simulink model "sim_3_twolink_task_control"  (R2021a)
settings: Solver=VariableStepAuto  StartTime=0.0  StopTime=10.0  RelTol=1e-3
values from neighbouring files (symbols this model uses):
  b1 = 0.01    [sim_params.m]    (also in sim_params_force.m)
  b2 = 0.01    [sim_params.m]    (also in sim_params_force.m)
  D = [zeros(n); eye(n)]    [control_comparison_script.m]    (also in gen_twolink_ss.m = reshape([0.0,0.0,0.0,0.0,0.0,0.0,0.0,0.0],[4,2]))
  g = 9.80665    [sim_params.m]    (also in sim_params_force.m)
  Klqr = lqr(A,B,Q,R)    [control_comparison_script.m]
  Kpp = place(A,B,p)    [control_comparison_script.m]
  L1x = 0.3    [sim_params.m]    (also in sim_params_force.m)
  L1y = 0.050    (= 0.05)    [sim_params.m]    (also in sim_params_force.m)
  L1z = 0.05    [sim_params.m]    (also in sim_params_force.m)
  L2x = 0.15    [sim_params.m]    (also in sim_params_force.m = 0.3)
  L2y = 0.05    [sim_params.m]    (also in sim_params_force.m)
  L2z = 0.05    [sim_params.m]    (also in sim_params_force.m)
  m1 = m1*1.25    [control_comparison_script.m]    (also in sim_params.m = 2.775; sim_params_force.m = 2.775)
  m2 = m2*1.25    [control_comparison_script.m]    (also in sim_params.m = 1.3875; sim_params_force.m = 2.775)
  max_joint_torque1 = 20    [sim_params.m]    (also in sim_params_force.m)
  max_joint_torque2 = 10    [sim_params.m]    (also in sim_params_force.m = 20)
  theta1_0 = 0    [sim_params.m]    (also in sim_params_force.m = 1.57079632679)
  theta1_dot_0 = 0    [sim_params.m]    (also in sim_params_force.m)
  theta2_0 = 0    [sim_params.m]    (also in sim_params_force.m = -1.57079632679)
  theta2_dot_0 = 0    [sim_params.m]    (also in sim_params_force.m)
undefined symbols (not defined in the file or in its folder): Kslide, lambda, Levenberg, Marquardt, phi, sigbuilder_block, X, Y, Z
libraries: sm_lib x11, nesl_utility x10, simulink x8, pid_lib x6, robotmaniplib x3, robotcorelib x1
(part 1 of 2)
settings Model: Creator=Petronas-Tareq  LastModifiedBy=Petronas-Tareq

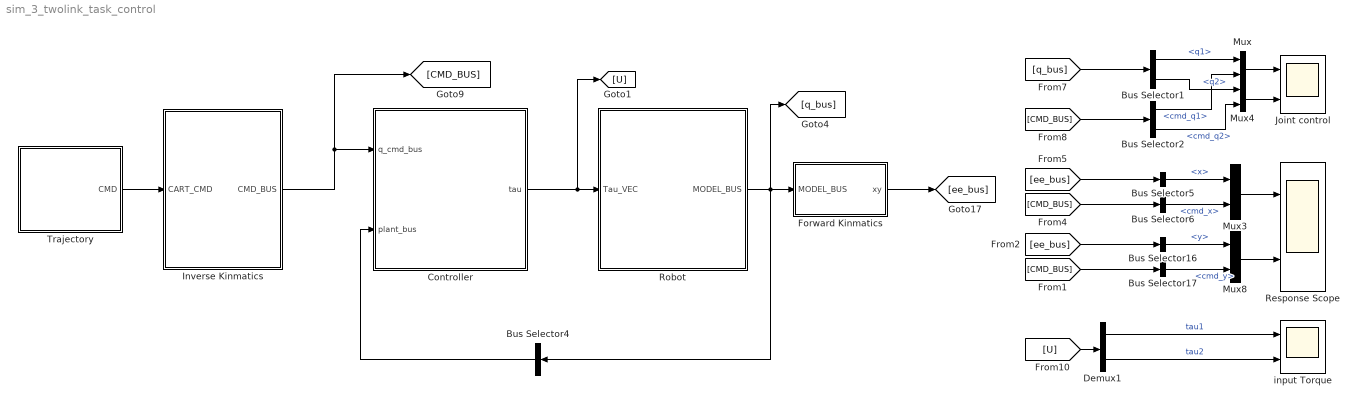
== system sim_3_twolink_task_control ==
  Bus Selector1 : BusSelector  OutputSignals=q1,q2
  Bus Selector16 : BusSelector  OutputSignals=y
  Bus Selector17 : BusSelector  OutputSignals=cmd_y
  Bus Selector2 : BusSelector  OutputSignals=cmd_q1,cmd_q2
  Bus Selector4 : BusSelector  OutputSignals=q1_dd,q2_dd,q1_d,q2_d,q1,q2  OutputAsBus=on
  Bus Selector5 : BusSelector  OutputSignals=x
  Bus Selector6 : BusSelector  OutputSignals=cmd_x
  Controller : Subsystem  Variant=on  VariantControlMode=label  LabelModeActiveChoice=PD_plus_gravity  PropagateVariantConditions=on
  Demux1 : Demux  Outputs=2
  Forward Kinmatics : Subsystem
  Inverse Kinmatics : Subsystem
  Joint control : Scope  NumInputPorts=2
  Mux{,3..4,8} (4 alike) : Mux  Inputs=2
  Response Scope : Scope  NumInputPorts=2
  Robot : Subsystem  Variant=on  VariantControlMode=label  LabelModeActiveChoice=Choice_1
  Trajectory : Subsystem  Variant=on  VariantControlMode=label  LabelModeActiveChoice=ramp
  input Torque : Scope  NumInputPorts=2
  wires:
  Trajectory/1(CMD) -> Inverse Kinmatics/1(CART_CMD)
  Robot/1(MODEL_BUS) -> Forward Kinmatics/1(MODEL_BUS), [q_bus], Bus Selector4/1
  Controller/1(tau) -> [U], Robot/1(Tau_VEC)
  Bus Selector4/1 -> Controller/2(plant_bus)
  Bus Selector2/1 -> Mux/2  "<cmd_q1>"
  Bus Selector1/2 -> Mux4/1  "<q2>"
  Mux4/1 -> Joint control/2
  [CMD_BUS] -> Bus Selector2/1
  Bus Selector1/1 -> Mux/1  "<q1>"
  Mux/1 -> Joint control/1
  Bus Selector2/2 -> Mux4/2  "<cmd_q2>"
  [q_bus] -> Bus Selector1/1
  Inverse Kinmatics/1(CMD_BUS) -> [CMD_BUS], Controller/1(q_cmd_bus)
  [ee_bus] -> Bus Selector5/1
  Bus Selector17/1 -> Mux8/2  "<cmd_y>"
  [U] -> Demux1/1
  [CMD_BUS] -> Bus Selector17/1
  Bus Selector16/1 -> Mux8/1  "<y>"
  Demux1/2 -> input Torque/2  "tau2"
  [ee_bus] -> Bus Selector16/1
  Demux1/1 -> input Torque/1  "tau1"
  Mux8/1 -> Response Scope/2
  Bus Selector6/1 -> Mux3/2  "<cmd_x>"
  [CMD_BUS] -> Bus Selector6/1
  Bus Selector5/1 -> Mux3/1  "<x>"
  Mux3/1 -> Response Scope/1
  Forward Kinmatics/1(xy) -> [ee_bus]

== system sim_3_twolink_task_control/Controller ==
  note: 1) Add Subsystem or Model blocks as valid variant choices.
      | 2) You cannot connect blocks at this level. At simulation, connectivity is automatically
      | determined, based on the active variant and port name matching.
  q_cmd_bus : Inport
  plant_bus : Inport  Port=2
  Incremental sliding mode Control : Subsystem  VariantControl=Sliding_mode_control
  "Inverse Dynamics control " : Subsystem  VariantControl=Inverse_dynamics_control
  LQR+D Control : Subsystem  VariantControl=LQR_D_control
  "PD-gravity Control " : Subsystem  VariantControl=PD_plus_gravity
  PID Control : Subsystem  VariantControl=PID_control
  Pole Placement+D Control : Subsystem  VariantControl=PolePlacement_D_control
  tau : Outport

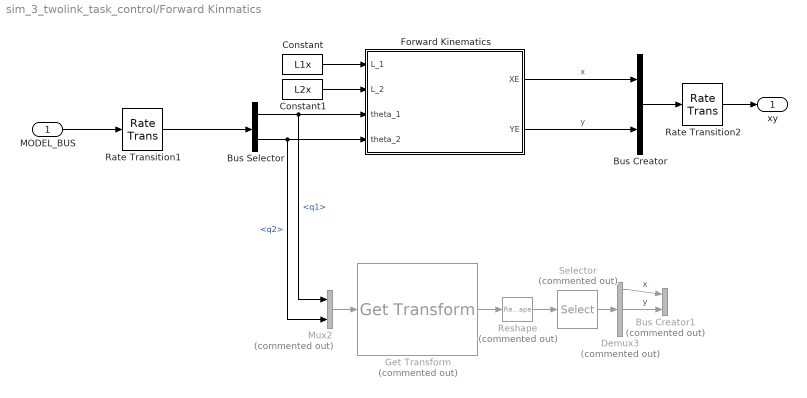
== system sim_3_twolink_task_control/Forward Kinmatics ==
  MODEL_BUS : Inport
  Bus Creator : BusCreator  Inputs=2
  Bus Creator1 : BusCreator  Commented=on  Inputs=2
  Bus Selector : BusSelector  OutputSignals=q1,q2
  Constant : Constant  Value=L1x
  Constant1 : Constant  Value=L2x
  Demux3 : Demux  Commented=on  Outputs=3
  Forward Kinematics : MATLAB Function  TreatAsAtomicUnit=on
  Get Transform : robotmaniplib/Get Transform  Commented=on  RigidBodyTree=RR_robot  SourceBody=end_effector  TargetBody=base  SimulateUsing=Interpreted execution
  Mux2 : Mux  Commented=on  Inputs=2
  Rate Transition1 : RateTransition  OutPortSampleTimeOpt=Inherit
  Rate Transition2 : RateTransition  OutPortSampleTimeOpt=Inherit
  Reshape : Reshape  Commented=on
  Selector : Selector  Commented=on  InputPortWidth=16  IndexOptions=Index vector (dialog)  Indices=[13:15]  OutputSizes=1
  xy : Outport
  wires:
  Forward Kinematics/2(YE) -> Bus Creator/2  "y"
  Forward Kinematics/1(XE) -> Bus Creator/1  "x"
  Bus Selector/1 -> Mux2/1, Forward Kinematics/3(theta_1)  "<q1>"
  MODEL_BUS/1 -> Rate Transition1/1
  Bus Selector/2 -> Mux2/2, Forward Kinematics/4(theta_2)  "<q2>"
  Constant/1 -> Forward Kinematics/1(L_1)
  Constant1/1 -> Forward Kinematics/2(L_2)
  Bus Creator/1 -> Rate Transition2/1
  Mux2/1 -> Get Transform/1
  Get Transform/1 -> Reshape/1
  Reshape/1 -> Selector/1
  Selector/1 -> Demux3/1
  Demux3/1 -> Bus Creator1/1  "x"
  Demux3/2 -> Bus Creator1/2  "y"
  Rate Transition2/1 -> xy/1
  Rate Transition1/1 -> Bus Selector/1

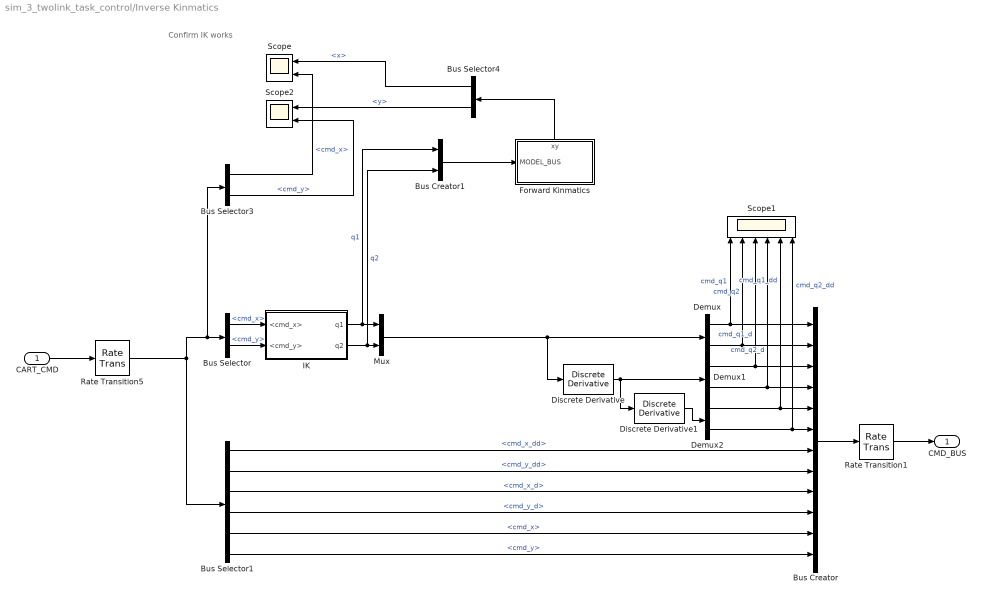
== system sim_3_twolink_task_control/Inverse Kinmatics ==
  note: Confirm IK works
  CART_CMD : Inport
  Bus Creator : BusCreator  Inputs=12
  Bus Creator1 : BusCreator  Inputs=2
  Bus Selector : BusSelector  OutputSignals=cmd_x,cmd_y
  Bus Selector1 : BusSelector  OutputSignals=cmd_x_dd,cmd_y_dd,cmd_x_d,cmd_y_d,cmd_x,cmd_y
  Bus Selector3 : BusSelector  OutputSignals=cmd_x,cmd_y
  Bus Selector4 : BusSelector  OutputSignals=x,y
  Demux : Demux  Outputs=2
  Demux1 : Demux  Outputs=2
  Demux2 : Demux  Outputs=2
  Discrete Derivative : simulink/Discrete/Discrete Derivative  gainval=1.0  ICPrevScaledInput=0.0  OutMin=[]  OutMax=[]  OutDataType=fixdt(1, 16)  OutScaling=2^-10  DoSatur=off
  Discrete Derivative1 : simulink/Discrete/Discrete Derivative  gainval=1.0  ICPrevScaledInput=0.0  OutMin=[]  OutMax=[]  OutDataType=fixdt(1, 16)  OutScaling=2^-10  DoSatur=off
  Forward Kinmatics : Subsystem
      settings: PortSchema="{\"entries\":[{\"content\":{\"sides\":[{\"content\":{\"connectorIds\":[\"In1\"]},\"type\":\"ConnectorPlacement.EquallySpacedRectSide\",\"uuid\":\"2c0f0405-b445-4922-82b0-9ed34ea6e343\"},{\"content\":{\"connectorIds\":[],\"side\":\"RIGHT\"},\"type\":\"ConnectorPlacement.EquallySpacedRectSide\",\"uuid\":\"91fea7c3-4850-470e-b524-5886f9b138cb\"},{\"content\":{\"connectorIds\":[\"Out1\"],\"side\":\"TOP\"},\"type\":\"ConnectorPlacement.EquallySpacedRectSide\",\"uuid\":\"51029b8b-093e-4a55-82a5-f93421c28d2e\"}]},\"type\":\"ConnectorPlacement.EquallySpacedConnector\",\"uuid\":\"843aee16-b8cd-4273-ac03-a5f22ed539be\"}],\"packageUris\":[\"http://schema.mathworks.com/mf0/Connector/R2020b\"],\"version\":\"1.0\"}"
  IK : Subsystem
  Mux : Mux  Inputs=2
  Rate Transition1 : RateTransition  OutPortSampleTimeOpt=Inherit
  Rate Transition5 : RateTransition  OutPortSampleTimeOpt=Inherit
  Scope : Scope  NumInputPorts=2
  Scope1 : Scope  NumInputPorts=6
  Scope2 : Scope  NumInputPorts=2
  CMD_BUS : Outport
  wires:
  Rate Transition5/1 -> Bus Selector3/1, Bus Selector/1, Bus Selector1/1
  Bus Creator/1 -> Rate Transition1/1
  Bus Selector1/1 -> Bus Creator/7  "<cmd_x_dd>"
  Bus Selector1/2 -> Bus Creator/8  "<cmd_y_dd>"
  Bus Selector1/3 -> Bus Creator/9  "<cmd_x_d>"
  Bus Selector1/4 -> Bus Creator/10  "<cmd_y_d>"
  Bus Selector1/5 -> Bus Creator/11  "<cmd_x>"
  Bus Selector1/6 -> Bus Creator/12  "<cmd_y>"
  Demux1/1 -> Scope1/3, Bus Creator/3  "cmd_q1_d"
  Demux2/2 -> Scope1/6, Bus Creator/6  "cmd_q2_dd"
  Demux1/2 -> Scope1/4, Bus Creator/4  "cmd_q2_d"
  Demux/1 -> Scope1/1, Bus Creator/1  "cmd_q1"
  Demux/2 -> Scope1/2, Bus Creator/2  "cmd_q2"
  Bus Selector/1 -> IK/1(<cmd_x>)  "<cmd_x>"
  Bus Selector/2 -> IK/2(<cmd_y>)  "<cmd_y>"
  IK/1(q1) -> Bus Creator1/1, Mux/1  "q1"
  IK/2(q2) -> Bus Creator1/2, Mux/2  "q2"
  Mux/1 -> Demux/1, Discrete Derivative/1
  Discrete Derivative/1 -> Demux1/1, Discrete Derivative1/1
  Demux2/1 -> Scope1/5, Bus Creator/5  "cmd_q1_dd"
  Discrete Derivative1/1 -> Demux2/1
  CART_CMD/1 -> Rate Transition5/1
  Rate Transition1/1 -> CMD_BUS/1
  Bus Creator1/1 -> Forward Kinmatics/1(MODEL_BUS)
  Forward Kinmatics/1(xy) -> Bus Selector4/1
  Bus Selector3/1 -> Scope/2  "<cmd_x>"
  Bus Selector4/1 -> Scope/1  "<x>"
  Bus Selector4/2 -> Scope2/1  "<y>"
  Bus Selector3/2 -> Scope2/2  "<cmd_y>"

== system sim_3_twolink_task_control/Robot ==
  note: 1) Add Subsystem or Model blocks as valid variant choices.
      | 2) You cannot connect blocks at this level. At simulation, connectivity is automatically
      | determined, based on the active variant and port name matching.
  Tau_VEC : Inport
  SIMSCAPE_MODEL : Subsystem  VariantControl=Choice_1
  SIMULINK_MODEL : Subsystem  VariantControl=Choice
  MODEL_BUS : Outport

== system sim_3_twolink_task_control/Trajectory ==
  note: 1) Add Subsystem or Model blocks as valid variant choices.
      | 2) You cannot connect blocks at this level. At simulation, connectivity is automatically
      | determined, based on the active variant and port name matching.
  Sinewave command : Subsystem  VariantControl=sinwave
  Step command : Subsystem  VariantControl=step
  ramp command : Subsystem  VariantControl=ramp
  CMD : Outport

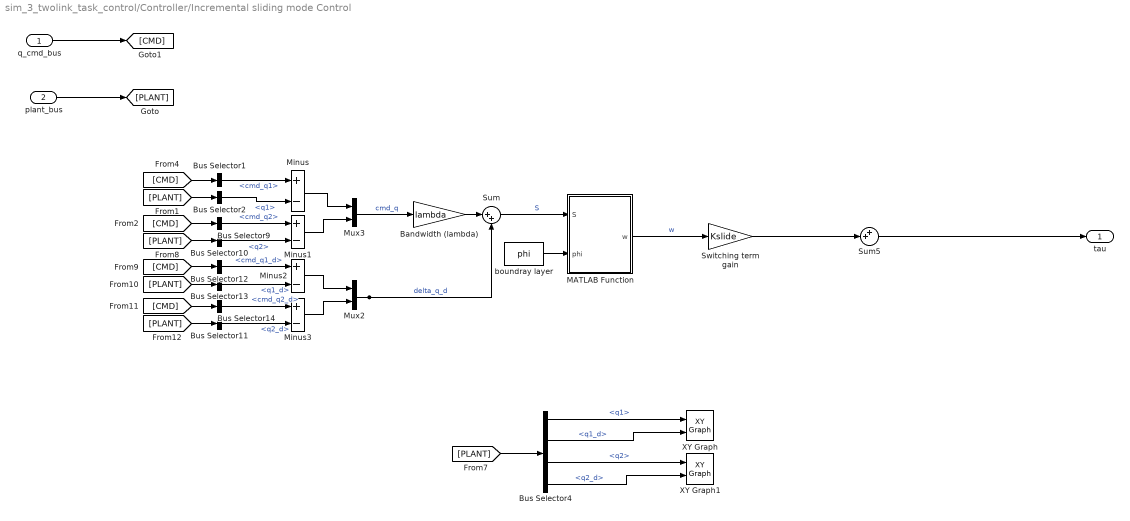
== system sim_3_twolink_task_control/Controller/Incremental sliding mode Control ==
  q_cmd_bus : Inport
  plant_bus : Inport  Port=2
  Bandwidth (lambda) : Gain  Gain=lambda
  Bus Selector1 : BusSelector  OutputSignals=cmd_q1
  Bus Selector10 : BusSelector  OutputSignals=q2
  Bus Selector11 : BusSelector  OutputSignals=q2_d
  Bus Selector12 : BusSelector  OutputSignals=cmd_q1_d
  Bus Selector13 : BusSelector  OutputSignals=q1_d
  Bus Selector14 : BusSelector  OutputSignals=cmd_q2_d
  Bus Selector2 : BusSelector  OutputSignals=q1
  Bus Selector4 : BusSelector  OutputSignals=q1,q1_d,q2,q2_d
  Bus Selector9 : BusSelector  OutputSignals=cmd_q2
  MATLAB Function : MATLAB Function  TreatAsAtomicUnit=on
  Minus{,1..3} (4 alike) : Sum  Inputs=+-
  Mux2 : Mux  Inputs=2
  Mux3 : Mux  Inputs=2
  Sum : Sum  Inputs=|++
  Sum5 : Sum  Inputs=++|
  Switching term gain : Gain  Gain=Kslide
  XY Graph : simulink/Sinks/XY Graph  xmin=-3  xmax=3  ymin=-3  ymax=3  st=-1
  XY Graph1 : simulink/Sinks/XY Graph  xmin=-3  xmax=3  ymin=-3  ymax=3  st=-1
  boundray layer : Constant  Value=phi
  tau : Outport
  wires:
  q_cmd_bus/1 -> [CMD]
  plant_bus/1 -> [PLANT]
  boundray layer/1 -> MATLAB Function/2(phi)
  [CMD] -> Bus Selector12/1
  Bus Selector1/1 -> Minus/1  "<cmd_q1>"
  [PLANT] -> Bus Selector13/1
  [PLANT] -> Bus Selector10/1
  [CMD] -> Bus Selector1/1
  Minus/1 -> Mux3/1
  [PLANT] -> Bus Selector11/1
  Minus3/1 -> Mux2/2
  [CMD] -> Bus Selector9/1
  Bus Selector12/1 -> Minus2/1  "<cmd_q1_d>"
  Bus Selector10/1 -> Minus1/2  "<q2>"
  Bus Selector2/1 -> Minus/2  "<q1>"
  Bus Selector9/1 -> Minus1/1  "<cmd_q2>"
  [PLANT] -> Bus Selector2/1
  Bus Selector11/1 -> Minus3/2  "<q2_d>"
  Bus Selector13/1 -> Minus2/2  "<q1_d>"
  Bus Selector14/1 -> Minus3/1  "<cmd_q2_d>"
  Minus2/1 -> Mux2/1
  [CMD] -> Bus Selector14/1
  Minus1/1 -> Mux3/2
  Sum/1 -> MATLAB Function/1(S)  "S"
  MATLAB Function/1(w) -> Switching term gain/1  "w"
  Switching term gain/1 -> Sum5/2
  Mux3/1 -> Bandwidth (lambda)/1  "cmd_q"
  Mux2/1 -> Sum/2  "delta_q_d"
  Bandwidth (lambda)/1 -> Sum/1
  Sum5/1 -> tau/1
  Bus Selector4/1 -> XY Graph/1  "<q1>"
  [PLANT] -> Bus Selector4/1
  Bus Selector4/2 -> XY Graph/2  "<q1_d>"
  Bus Selector4/3 -> XY Graph1/1  "<q2>"
  Bus Selector4/4 -> XY Graph1/2  "<q2_d>"

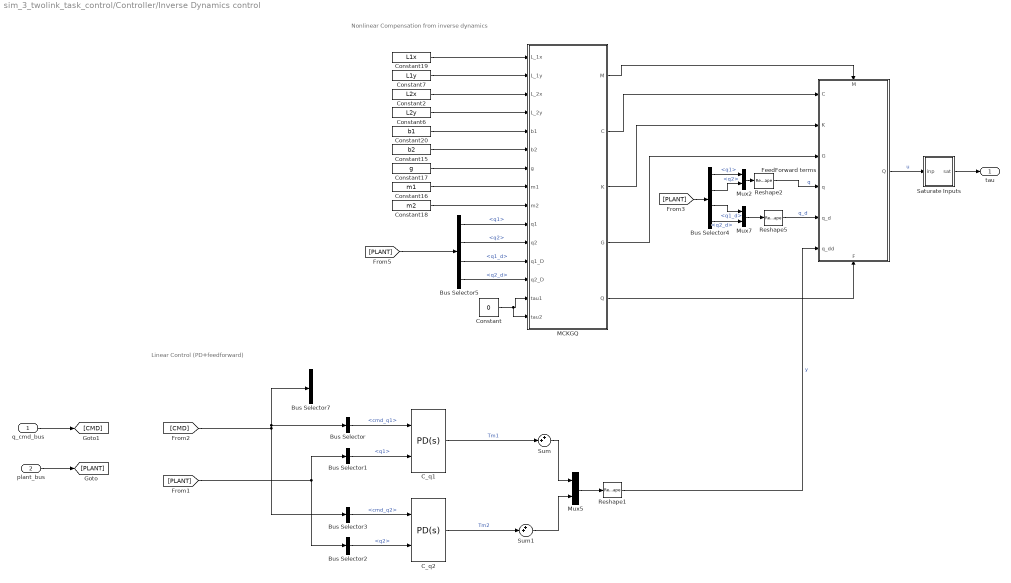
== system sim_3_twolink_task_control/Controller/Inverse Dynamics control  ==
  note: Nonlinear Compensation from inverse dynamics
  note: Linear Control (PD+feedforward)
  q_cmd_bus : Inport
  plant_bus : Inport  Port=2
  Bus Selector : BusSelector  OutputSignals=cmd_q1
  Bus Selector1 : BusSelector  OutputSignals=q1
  Bus Selector2 : BusSelector  OutputSignals=q2
  Bus Selector3 : BusSelector  OutputSignals=cmd_q2
  Bus Selector4 : BusSelector  OutputSignals=q1,q2,q1_d,q2_d
  Bus Selector5 : BusSelector  OutputSignals=q1,q2,q1_d,q2_d
  Bus Selector7 : BusSelector  OutputSignals=cmd_q1_dd,cmd_q2_dd
  C_q1 : pid_lib/PID Controller (2DOF)  Controller=PD  Form=Parallel  TimeDomain=Continuous-time  UseExternalTs=off  SampleTime=-1  IntegratorMethod=Forward Euler  FilterMethod=Forward Euler  ControllerParametersSource=internal  P=400  I=20  D=40  UseFilter=on  N=100  b=1  c=1  TunerSelectOption=Transfer Function Based (PID Tuner App)  InitialConditionSource=internal  InitialConditionForIntegrator=0  InitialConditionForFilter=0  DifferentiatorICPrevScaledInput=0  ExternalReset=none  TrackingMode=off  Kt=1  LimitOutput=on  SatLimitsSource=internal  UpperSaturationLimit=max_joint_torque1  LowerSaturationLimit=-max_joint_torque1  LinearizeAsGain=on  AntiWindupMode=none  Kb=1  POutMin=[]  POutMax=[]  IOutMin=[]  IOutMax=[]  DOutMin=[]  DOutMax=[]  NOutMin=[]  NOutMax=[]  bOutMin=[]  bOutMax=[]  cOutMin=[]  cOutMax=[]  SumOutMin=[]  SumOutMax=[]  SaturationOutMin=[]  SaturationOutMax=[]  PParamMin=[]  PParamMax=[]  IParamMin=[]  IParamMax=[]  DParamMin=[]  DParamMax=[]  NParamMin=[]  NParamMax=[]  bParamMin=[]  bParamMax=[]  cParamMin=[]  cParamMax=[]  KbParamMin=[]  KbParamMax=[]  KtParamMin=[]  KtParamMax=[]  KbOutMin=[]  KbOutMax=[]  KtOutMin=[]  KtOutMax=[]  IntegratorOutMin=[]  IntegratorOutMax=[]  FilterOutMin=[]  FilterOutMax=[]  SumI1OutMin=[]  SumI1OutMax=[]  SumI2OutMin=[]  SumI2OutMax=[]  SumI3OutMin=[]  SumI3OutMax=[]  SumI4OutMin=[]  SumI4OutMax=[]  SumDOutMin=[]  SumDOutMax=[]  Sum1OutMin=[]  Sum1OutMax=[]  Sum2OutMin=[]  Sum2OutMax=[]  Sum3OutMin=[]  Sum3OutMax=[]  DifferentiatorOutMin=[]  DifferentiatorOutMax=[]  FilterDiffOutCoefMin=[]  FilterDiffOutCoefMax=[]  ReciprocalOutMin=[]  ReciprocalOutMax=[]  SumDenOutMin=[]  SumDenOutMax=[]  SumNumOutMin=[]  SumNumOutMax=[]  DivideOutMin=[]  DivideOutMax=[]  UdiffTsProdOutMin=[]  UdiffTsProdOutMax=[]  NTsProdOutMin=[]  NTsProdOutMax=[]  UintegralTsProdOutMin=[]  UintegralTsProdOutMax=[]  UngainTsProdOutMin=[]  UngainTsProdOutMax=[]  IntegratorContinuousStateAttributes=''  IntegratorStateMustResolveToSignalObject=off  IntegratorRTWStateStorageClass=Auto  FilterContinuousStateAttributes=''  FilterStateMustResolveToSignalObject=off  FilterRTWStateStorageClass=Auto  ParallelPVariant=InternalParameters  IdealPVariant=Disabled  IVariant=Disabled  DVariant=InternalParameters  bVariant=InternalParameters  cVariant=InternalParameters  IntegratorVariant=Disabled  SatVariant=Enabled  AWVariant=Disabled  PCopyVariant=Disabled  TRVariant=Disabled  FdbkBlocksVariant=Forward  IdealPFdbkVariant=Disabled  SatFdbkVariant=Disabled  DerivativeFilterVariant=ContFilter  NVariant=InternalParameters  NCopyVariant=Disabled  FilterICVariant=InternalICsFilter  IntegratorICVariant=Disabled  ExternalResetVariant=Disabled  TRSumVariant=Passthrough  SumFdbkVariant=Disabled  SumVariant=Sum_PD  TsampFilterVariant=InternalTs  TsampNgainVariant=Passthrough  TsampIntegralVariant=Disabled_SignalSpec  ExternalSaturationOutDataTypeStr=Inherit: Same as second input
      settings: SourceProductBaseCode=SL
  C_q2 : pid_lib/PID Controller (2DOF)  Controller=PD  Form=Parallel  TimeDomain=Continuous-time  UseExternalTs=off  SampleTime=-1  IntegratorMethod=Forward Euler  FilterMethod=Forward Euler  ControllerParametersSource=internal  P=200  I=20  D=35  UseFilter=on  N=100  b=1  c=1  TunerSelectOption=Transfer Function Based (PID Tuner App)  InitialConditionSource=internal  InitialConditionForIntegrator=0  InitialConditionForFilter=0  DifferentiatorICPrevScaledInput=0  ExternalReset=none  TrackingMode=off  Kt=1  LimitOutput=on  SatLimitsSource=internal  UpperSaturationLimit=max_joint_torque2  LowerSaturationLimit=-max_joint_torque2  LinearizeAsGain=on  AntiWindupMode=none  Kb=1  POutMin=[]  POutMax=[]  IOutMin=[]  IOutMax=[]  DOutMin=[]  DOutMax=[]  NOutMin=[]  NOutMax=[]  bOutMin=[]  bOutMax=[]  cOutMin=[]  cOutMax=[]  SumOutMin=[]  SumOutMax=[]  SaturationOutMin=[]  SaturationOutMax=[]  PParamMin=[]  PParamMax=[]  IParamMin=[]  IParamMax=[]  DParamMin=[]  DParamMax=[]  NParamMin=[]  NParamMax=[]  bParamMin=[]  bParamMax=[]  cParamMin=[]  cParamMax=[]  KbParamMin=[]  KbParamMax=[]  KtParamMin=[]  KtParamMax=[]  KbOutMin=[]  KbOutMax=[]  KtOutMin=[]  KtOutMax=[]  IntegratorOutMin=[]  IntegratorOutMax=[]  FilterOutMin=[]  FilterOutMax=[]  SumI1OutMin=[]  SumI1OutMax=[]  SumI2OutMin=[]  SumI2OutMax=[]  SumI3OutMin=[]  SumI3OutMax=[]  SumI4OutMin=[]  SumI4OutMax=[]  SumDOutMin=[]  SumDOutMax=[]  Sum1OutMin=[]  Sum1OutMax=[]  Sum2OutMin=[]  Sum2OutMax=[]  Sum3OutMin=[]  Sum3OutMax=[]  DifferentiatorOutMin=[]  DifferentiatorOutMax=[]  FilterDiffOutCoefMin=[]  FilterDiffOutCoefMax=[]  ReciprocalOutMin=[]  ReciprocalOutMax=[]  SumDenOutMin=[]  SumDenOutMax=[]  SumNumOutMin=[]  SumNumOutMax=[]  DivideOutMin=[]  DivideOutMax=[]  UdiffTsProdOutMin=[]  UdiffTsProdOutMax=[]  NTsProdOutMin=[]  NTsProdOutMax=[]  UintegralTsProdOutMin=[]  UintegralTsProdOutMax=[]  UngainTsProdOutMin=[]  UngainTsProdOutMax=[]  IntegratorContinuousStateAttributes=''  IntegratorStateMustResolveToSignalObject=off  IntegratorRTWStateStorageClass=Auto  FilterContinuousStateAttributes=''  FilterStateMustResolveToSignalObject=off  FilterRTWStateStorageClass=Auto  ParallelPVariant=InternalParameters  IdealPVariant=Disabled  IVariant=Disabled  DVariant=InternalParameters  bVariant=InternalParameters  cVariant=InternalParameters  IntegratorVariant=Disabled  SatVariant=Enabled  AWVariant=Disabled  PCopyVariant=Disabled  TRVariant=Disabled  FdbkBlocksVariant=Forward  IdealPFdbkVariant=Disabled  SatFdbkVariant=Disabled  DerivativeFilterVariant=ContFilter  NVariant=InternalParameters  NCopyVariant=Disabled  FilterICVariant=InternalICsFilter  IntegratorICVariant=Disabled  ExternalResetVariant=Disabled  TRSumVariant=Passthrough  SumFdbkVariant=Disabled  SumVariant=Sum_PD  TsampFilterVariant=InternalTs  TsampNgainVariant=Passthrough  TsampIntegralVariant=Disabled_SignalSpec  ExternalSaturationOutDataTypeStr=Inherit: Same as second input
      settings: SourceProductBaseCode=SL
  Constant : Constant  Value=0
  Constant15 : Constant  Value=b2
  Constant16 : Constant  Value=m1
  Constant17 : Constant  Value=g
  Constant18 : Constant  Value=m2
  Constant19 : Constant  Value=L1x
  Constant2 : Constant  Value=L2x
  Constant20 : Constant  Value=b1
  Constant6 : Constant  Value=L2y
  Constant7 : Constant  Value=L1y
  FeedForward terms : Subsystem
      settings: PortSchema="{\"entries\":[{\"content\":{\"sides\":[{\"content\":{\"connectorIds\":[\"In1\",\"In2\",\"In3\",\"In4\",\"In5\",\"In6\"]},\"type\":\"ConnectorPlacement.EquallySpacedRectSide\",\"uuid\":\"236e7a2f-027c-4887-b3e9-bc0e11a59ec6\"},{\"content\":{\"connectorIds\":[\"Out1\"],\"side\":\"RIGHT\"},\"type\":\"ConnectorPlacement.EquallySpacedRectSide\",\"uuid\":\"0b727d96-7650-4ea0-95ac-5fb1bad7af10\"},{\"content\":{\"connectorIds\":[\"In7\"],\"side\":\"TOP\"},\"type\":\"ConnectorPlacement.EquallySpacedRectSide\",\"uuid\":\"19d9c8c6-ae7e-49b4-b718-472bd3040569\"},{\"content\":{\"connectorIds\":[\"In8\"],\"side\":\"BOTTOM\"},\"type\":\"ConnectorPlacement.EquallySpacedRectSide\",\"uuid\":\"734f5953-872d-4718-8798-69ea98da43e1\"}]},\"type\":\"ConnectorPlacement.EquallySpacedConnector\",\"uuid\":\"f4b93fea-e2dd-47f1-bf2a-cf2dec03adb9\"}],\"packageUris\":[\"http://schema.mathworks.com/mf0/Connector/R2020b\"],\"version\":\"1.0\"}"
  MCKGQ : MATLAB Function  TreatAsAtomicUnit=on
  Mux2 : Mux  Inputs=2
  Mux5 : Mux  Inputs=2
  Mux7 : Mux  Inputs=2
  Reshape1 : Reshape  OutputDimensionality=Column vector (2-D)
  Reshape2 : Reshape  OutputDimensionality=Column vector (2-D)
  Reshape5 : Reshape  OutputDimensionality=Column vector (2-D)
  Saturate Inputs : Subsystem
  Sum : Sum  Inputs=++|
  Sum1 : Sum  Inputs=++|
  tau : Outport
  wires:
  C_q1/1 -> Sum/2  "Tm1"
  q_cmd_bus/1 -> [CMD]
  plant_bus/1 -> [PLANT]
  Bus Selector2/1 -> C_q2/2  "<q2>"
  Bus Selector3/1 -> C_q2/1  "<cmd_q2>"
  Bus Selector1/1 -> C_q1/2  "<q1>"
  Bus Selector/1 -> C_q1/1  "<cmd_q1>"
  [PLANT] -> Bus Selector1/1, Bus Selector2/1
  Bus Selector5/4 -> MCKGQ/13(q2_D)  "<q2_d>"
  Bus Selector5/3 -> MCKGQ/12(q1_D)  "<q1_d>"
  Bus Selector5/1 -> MCKGQ/10(q1)  "<q1>"
  [PLANT] -> Bus Selector5/1
  Bus Selector5/2 -> MCKGQ/11(q2)  "<q2>"
  Mux5/1 -> Reshape1/1
  FeedForward terms/1(Q) -> Saturate Inputs/1(inp)  "u"
  [CMD] -> Bus Selector7/1, Bus Selector/1, Bus Selector3/1
  Sum/1 -> Mux5/1
  C_q2/1 -> Sum1/2  "Tm2"
  Sum1/1 -> Mux5/2
  [PLANT] -> Bus Selector4/1
  Bus Selector4/3 -> Mux7/1  "<q1_d>"
  Bus Selector4/4 -> Mux7/2  "<q2_d>"
  Mux7/1 -> Reshape5/1
  Reshape5/1 -> FeedForward terms/5(q_d)  "q_d"
  Reshape1/1 -> FeedForward terms/6(q_dd)  "y"
  MCKGQ/2(C) -> FeedForward terms/1(C)
  MCKGQ/3(K) -> FeedForward terms/2(K)
  MCKGQ/4(G) -> FeedForward terms/3(G)
  Bus Selector4/1 -> Mux2/1  "<q1>"
  Bus Selector4/2 -> Mux2/2  "<q2>"
  Mux2/1 -> Reshape2/1
  Reshape2/1 -> FeedForward terms/4(q)  "q"
  MCKGQ/5(Q) -> FeedForward terms/8(F)
  Constant/1 -> MCKGQ/14(tau1), MCKGQ/15(tau2)
  MCKGQ/1(M) -> FeedForward terms/7(M)
  Constant7/1 -> MCKGQ/2(L_1y)
  Constant2/1 -> MCKGQ/3(L_2x)
  Constant6/1 -> MCKGQ/4(L_2y)
  Constant20/1 -> MCKGQ/5(b1)
  Constant15/1 -> MCKGQ/6(b2)
  Constant17/1 -> MCKGQ/7(g)
  Constant16/1 -> MCKGQ/8(m1)
  Constant18/1 -> MCKGQ/9(m2)
  Constant19/1 -> MCKGQ/1(L_1x)
  Saturate Inputs/1(sat) -> tau/1

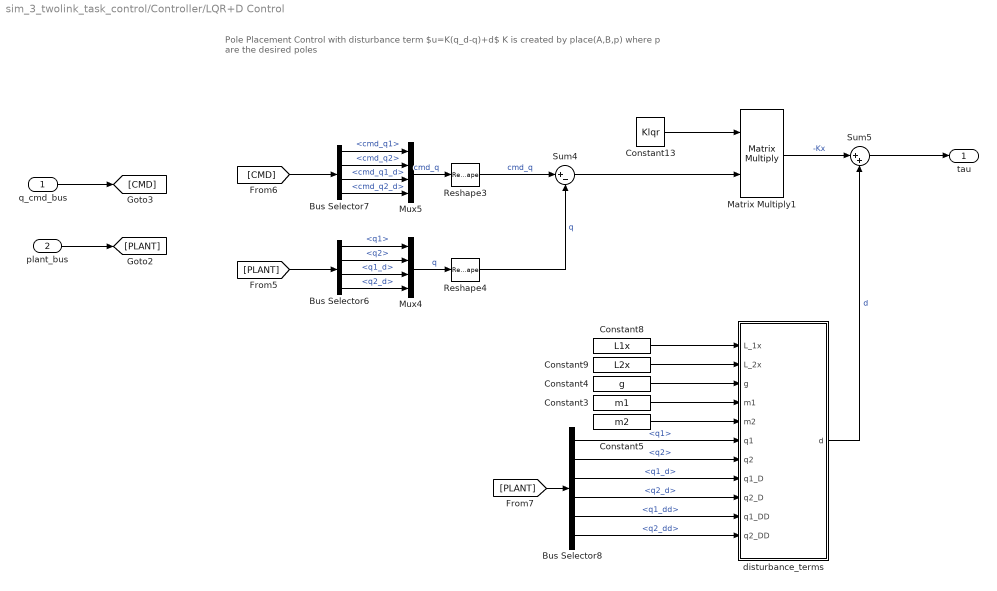
== system sim_3_twolink_task_control/Controller/LQR+D Control ==
  note: Pole Placement Control with disturbance term
      | $u=K(q_d-q)+d$
      | K is created by place(A,B,p) where p are the desired poles
  q_cmd_bus : Inport
  plant_bus : Inport  Port=2
  Bus Selector6 : BusSelector  OutputSignals=q1,q2,q1_d,q2_d
  Bus Selector7 : BusSelector  OutputSignals=cmd_q1,cmd_q2,cmd_q1_d,cmd_q2_d
  Bus Selector8 : BusSelector  OutputSignals=q1,q2,q1_d,q2_d,q1_dd,q2_dd
  Constant13 : Constant  Value=Klqr  VectorParams1D=off
  Constant3 : Constant  Value=m1
  Constant4 : Constant  Value=g
  Constant5 : Constant  Value=m2
  Constant8 : Constant  Value=L1x
  Constant9 : Constant  Value=L2x
  Matrix Multiply1 : Product  Multiplication=Matrix(*)
  Mux4 : Mux
  Mux5 : Mux
  Reshape3 : Reshape  OutputDimensionality=Column vector (2-D)
  Reshape4 : Reshape  OutputDimensionality=Column vector (2-D)
  Sum4 : Sum  Inputs=|+-
  Sum5 : Sum  Inputs=|++
  disturbance_terms : MATLAB Function  TreatAsAtomicUnit=on
  tau : Outport
  wires:
  Bus Selector6/2 -> Mux4/2  "<q2>"
  Bus Selector6/1 -> Mux4/1  "<q1>"
  Mux4/1 -> Reshape4/1  "q"
  q_cmd_bus/1 -> [CMD]
  plant_bus/1 -> [PLANT]
  Mux5/1 -> Reshape3/1  "cmd_q"
  Bus Selector6/3 -> Mux4/3  "<q1_d>"
  [PLANT] -> Bus Selector6/1
  Bus Selector6/4 -> Mux4/4  "<q2_d>"
  Reshape3/1 -> Sum4/1  "cmd_q"
  Reshape4/1 -> Sum4/2  "q"
  Matrix Multiply1/1 -> Sum5/1  "-Kx"
  Sum4/1 -> Matrix Multiply1/2
  Bus Selector7/1 -> Mux5/1  "<cmd_q1>"
  Bus Selector7/2 -> Mux5/2  "<cmd_q2>"
  Bus Selector7/3 -> Mux5/3  "<cmd_q1_d>"
  Constant13/1 -> Matrix Multiply1/1
  Bus Selector7/4 -> Mux5/4  "<cmd_q2_d>"
  [CMD] -> Bus Selector7/1
  Sum5/1 -> tau/1
  disturbance_terms/1(d) -> Sum5/2  "d"
  [PLANT] -> Bus Selector8/1
  Bus Selector8/1 -> disturbance_terms/6(q1)  "<q1>"
  Bus Selector8/2 -> disturbance_terms/7(q2)  "<q2>"
  Bus Selector8/3 -> disturbance_terms/8(q1_D)  "<q1_d>"
  Bus Selector8/4 -> disturbance_terms/9(q2_D)  "<q2_d>"
  Bus Selector8/5 -> disturbance_terms/10(q1_DD)  "<q1_dd>"
  Bus Selector8/6 -> disturbance_terms/11(q2_DD)  "<q2_dd>"
  Constant8/1 -> disturbance_terms/1(L_1x)
  Constant9/1 -> disturbance_terms/2(L_2x)
  Constant4/1 -> disturbance_terms/3(g)
  Constant3/1 -> disturbance_terms/4(m1)
  Constant5/1 -> disturbance_terms/5(m2)

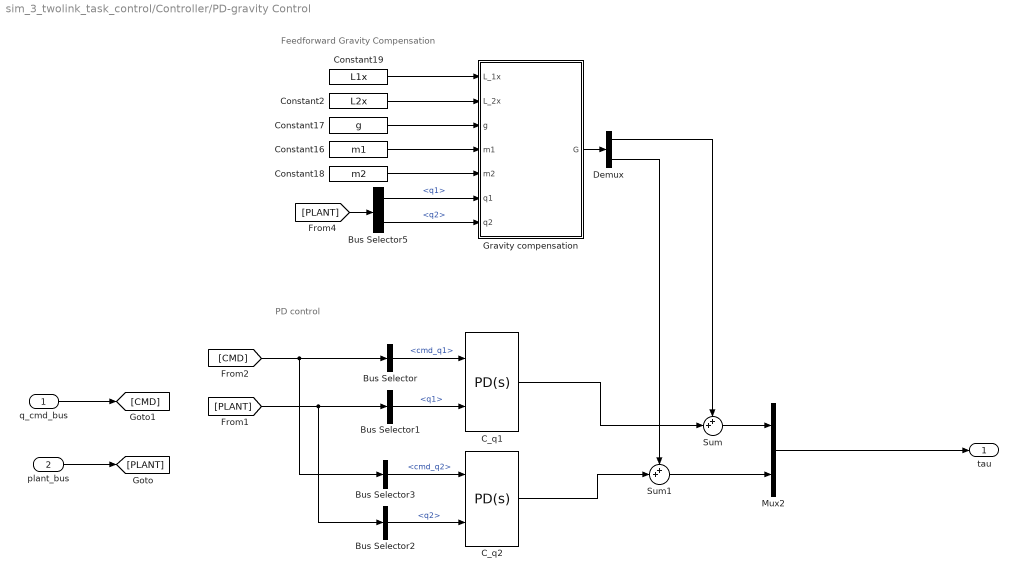
== system sim_3_twolink_task_control/Controller/PD-gravity Control  ==
  note: Feedforward Gravity Compensation
  note: PD control
  q_cmd_bus : Inport
  plant_bus : Inport  Port=2
  Bus Selector : BusSelector  OutputSignals=cmd_q1
  Bus Selector1 : BusSelector  OutputSignals=q1
  Bus Selector2 : BusSelector  OutputSignals=q2
  Bus Selector3 : BusSelector  OutputSignals=cmd_q2
  Bus Selector5 : BusSelector  OutputSignals=q1,q2
  C_q1 : pid_lib/PID Controller (2DOF)  Controller=PD  Form=Parallel  TimeDomain=Continuous-time  UseExternalTs=off  SampleTime=-1  IntegratorMethod=Forward Euler  FilterMethod=Forward Euler  ControllerParametersSource=internal  P=15  I=15  D=3  UseFilter=on  N=100  b=1  c=1  TunerSelectOption=Transfer Function Based (PID Tuner App)  InitialConditionSource=internal  InitialConditionForIntegrator=0  InitialConditionForFilter=0  DifferentiatorICPrevScaledInput=0  ExternalReset=none  TrackingMode=off  Kt=1  LimitOutput=off  SatLimitsSource=internal  UpperSaturationLimit=max_joint_torque1  LowerSaturationLimit=-max_joint_torque1  LinearizeAsGain=on  AntiWindupMode=none  Kb=1  POutMin=[]  POutMax=[]  IOutMin=[]  IOutMax=[]  DOutMin=[]  DOutMax=[]  NOutMin=[]  NOutMax=[]  bOutMin=[]  bOutMax=[]  cOutMin=[]  cOutMax=[]  SumOutMin=[]  SumOutMax=[]  SaturationOutMin=[]  SaturationOutMax=[]  PParamMin=[]  PParamMax=[]  IParamMin=[]  IParamMax=[]  DParamMin=[]  DParamMax=[]  NParamMin=[]  NParamMax=[]  bParamMin=[]  bParamMax=[]  cParamMin=[]  cParamMax=[]  KbParamMin=[]  KbParamMax=[]  KtParamMin=[]  KtParamMax=[]  KbOutMin=[]  KbOutMax=[]  KtOutMin=[]  KtOutMax=[]  IntegratorOutMin=[]  IntegratorOutMax=[]  FilterOutMin=[]  FilterOutMax=[]  SumI1OutMin=[]  SumI1OutMax=[]  SumI2OutMin=[]  SumI2OutMax=[]  SumI3OutMin=[]  SumI3OutMax=[]  SumI4OutMin=[]  SumI4OutMax=[]  SumDOutMin=[]  SumDOutMax=[]  Sum1OutMin=[]  Sum1OutMax=[]  Sum2OutMin=[]  Sum2OutMax=[]  Sum3OutMin=[]  Sum3OutMax=[]  DifferentiatorOutMin=[]  DifferentiatorOutMax=[]  FilterDiffOutCoefMin=[]  FilterDiffOutCoefMax=[]  ReciprocalOutMin=[]  ReciprocalOutMax=[]  SumDenOutMin=[]  SumDenOutMax=[]  SumNumOutMin=[]  SumNumOutMax=[]  DivideOutMin=[]  DivideOutMax=[]  UdiffTsProdOutMin=[]  UdiffTsProdOutMax=[]  NTsProdOutMin=[]  NTsProdOutMax=[]  UintegralTsProdOutMin=[]  UintegralTsProdOutMax=[]  UngainTsProdOutMin=[]  UngainTsProdOutMax=[]  IntegratorContinuousStateAttributes=''  IntegratorStateMustResolveToSignalObject=off  IntegratorRTWStateStorageClass=Auto  FilterContinuousStateAttributes=''  FilterStateMustResolveToSignalObject=off  FilterRTWStateStorageClass=Auto  ParallelPVariant=InternalParameters  IdealPVariant=Disabled  IVariant=Disabled  DVariant=InternalParameters  bVariant=InternalParameters  cVariant=InternalParameters  IntegratorVariant=Disabled  SatVariant=Disabled  AWVariant=Disabled  PCopyVariant=Disabled  TRVariant=Disabled  FdbkBlocksVariant=Forward  IdealPFdbkVariant=Disabled  SatFdbkVariant=Disabled  DerivativeFilterVariant=ContFilter  NVariant=InternalParameters  NCopyVariant=Disabled  FilterICVariant=InternalICsFilter  IntegratorICVariant=Disabled  ExternalResetVariant=Disabled  TRSumVariant=Passthrough  SumFdbkVariant=Disabled  SumVariant=Sum_PD  TsampFilterVariant=InternalTs  TsampNgainVariant=Passthrough  TsampIntegralVariant=Disabled_SignalSpec  ExternalSaturationOutDataTypeStr=Inherit: Same as second input
      settings: SourceProductBaseCode=SL
  C_q2 : pid_lib/PID Controller (2DOF)  Controller=PD  Form=Parallel  TimeDomain=Continuous-time  UseExternalTs=off  SampleTime=-1  IntegratorMethod=Forward Euler  FilterMethod=Forward Euler  ControllerParametersSource=internal  P=7  I=5  D=0.8  UseFilter=on  N=100  b=1  c=1  TunerSelectOption=Transfer Function Based (PID Tuner App)  InitialConditionSource=internal  InitialConditionForIntegrator=0  InitialConditionForFilter=0  DifferentiatorICPrevScaledInput=0  ExternalReset=none  TrackingMode=off  Kt=1  LimitOutput=off  SatLimitsSource=internal  UpperSaturationLimit=max_joint_torque2  LowerSaturationLimit=-max_joint_torque2  LinearizeAsGain=on  AntiWindupMode=none  Kb=1  POutMin=[]  POutMax=[]  IOutMin=[]  IOutMax=[]  DOutMin=[]  DOutMax=[]  NOutMin=[]  NOutMax=[]  bOutMin=[]  bOutMax=[]  cOutMin=[]  cOutMax=[]  SumOutMin=[]  SumOutMax=[]  SaturationOutMin=[]  SaturationOutMax=[]  PParamMin=[]  PParamMax=[]  IParamMin=[]  IParamMax=[]  DParamMin=[]  DParamMax=[]  NParamMin=[]  NParamMax=[]  bParamMin=[]  bParamMax=[]  cParamMin=[]  cParamMax=[]  KbParamMin=[]  KbParamMax=[]  KtParamMin=[]  KtParamMax=[]  KbOutMin=[]  KbOutMax=[]  KtOutMin=[]  KtOutMax=[]  IntegratorOutMin=[]  IntegratorOutMax=[]  FilterOutMin=[]  FilterOutMax=[]  SumI1OutMin=[]  SumI1OutMax=[]  SumI2OutMin=[]  SumI2OutMax=[]  SumI3OutMin=[]  SumI3OutMax=[]  SumI4OutMin=[]  SumI4OutMax=[]  SumDOutMin=[]  SumDOutMax=[]  Sum1OutMin=[]  Sum1OutMax=[]  Sum2OutMin=[]  Sum2OutMax=[]  Sum3OutMin=[]  Sum3OutMax=[]  DifferentiatorOutMin=[]  DifferentiatorOutMax=[]  FilterDiffOutCoefMin=[]  FilterDiffOutCoefMax=[]  ReciprocalOutMin=[]  ReciprocalOutMax=[]  SumDenOutMin=[]  SumDenOutMax=[]  SumNumOutMin=[]  SumNumOutMax=[]  DivideOutMin=[]  DivideOutMax=[]  UdiffTsProdOutMin=[]  UdiffTsProdOutMax=[]  NTsProdOutMin=[]  NTsProdOutMax=[]  UintegralTsProdOutMin=[]  UintegralTsProdOutMax=[]  UngainTsProdOutMin=[]  UngainTsProdOutMax=[]  IntegratorContinuousStateAttributes=''  IntegratorStateMustResolveToSignalObject=off  IntegratorRTWStateStorageClass=Auto  FilterContinuousStateAttributes=''  FilterStateMustResolveToSignalObject=off  FilterRTWStateStorageClass=Auto  ParallelPVariant=InternalParameters  IdealPVariant=Disabled  IVariant=Disabled  DVariant=InternalParameters  bVariant=InternalParameters  cVariant=InternalParameters  IntegratorVariant=Disabled  SatVariant=Disabled  AWVariant=Disabled  PCopyVariant=Disabled  TRVariant=Disabled  FdbkBlocksVariant=Forward  IdealPFdbkVariant=Disabled  SatFdbkVariant=Disabled  DerivativeFilterVariant=ContFilter  NVariant=InternalParameters  NCopyVariant=Disabled  FilterICVariant=InternalICsFilter  IntegratorICVariant=Disabled  ExternalResetVariant=Disabled  TRSumVariant=Passthrough  SumFdbkVariant=Disabled  SumVariant=Sum_PD  TsampFilterVariant=InternalTs  TsampNgainVariant=Passthrough  TsampIntegralVariant=Disabled_SignalSpec  ExternalSaturationOutDataTypeStr=Inherit: Same as second input
      settings: SourceProductBaseCode=SL
  Constant16 : Constant  Value=m1
  Constant17 : Constant  Value=g
  Constant18 : Constant  Value=m2
  Constant19 : Constant  Value=L1x
  Constant2 : Constant  Value=L2x
  Demux : Demux  Outputs=2
  Gravity compensation : MATLAB Function  TreatAsAtomicUnit=on
  Mux2 : Mux  Inputs=2
  Sum : Sum  Inputs=++|
  Sum1 : Sum  Inputs=++|
  tau : Outport
  wires:
  Sum/1 -> Mux2/1
  Sum1/1 -> Mux2/2
  q_cmd_bus/1 -> [CMD]
  plant_bus/1 -> [PLANT]
  Bus Selector5/1 -> Gravity compensation/6(q1)  "<q1>"
  [PLANT] -> Bus Selector5/1
  Bus Selector5/2 -> Gravity compensation/7(q2)  "<q2>"
  Gravity compensation/1(G) -> Demux/1
  Demux/1 -> Sum/1
  Demux/2 -> Sum1/1
  C_q2/1 -> Sum1/2
  [CMD] -> Bus Selector3/1, Bus Selector/1
  [PLANT] -> Bus Selector2/1, Bus Selector1/1
  Bus Selector1/1 -> C_q1/2  "<q1>"
  Bus Selector2/1 -> C_q2/2  "<q2>"
  Bus Selector3/1 -> C_q2/1  "<cmd_q2>"
  Bus Selector/1 -> C_q1/1  "<cmd_q1>"
  C_q1/1 -> Sum/2
  Constant19/1 -> Gravity compensation/1(L_1x)
  Constant2/1 -> Gravity compensation/2(L_2x)
  Constant17/1 -> Gravity compensation/3(g)
  Constant16/1 -> Gravity compensation/4(m1)
  Constant18/1 -> Gravity compensation/5(m2)
  Mux2/1 -> tau/1

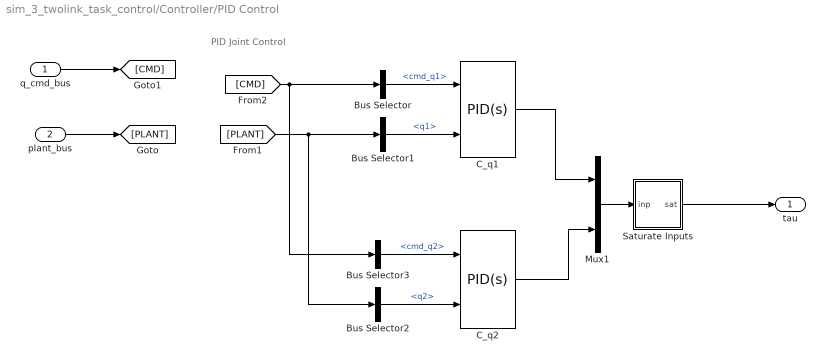
== system sim_3_twolink_task_control/Controller/PID Control ==
  note: PID Joint Control
  q_cmd_bus : Inport
  plant_bus : Inport  Port=2
  Bus Selector : BusSelector  OutputSignals=cmd_q1
  Bus Selector1 : BusSelector  OutputSignals=q1
  Bus Selector2 : BusSelector  OutputSignals=q2
  Bus Selector3 : BusSelector  OutputSignals=cmd_q2
  C_q1 : pid_lib/PID Controller (2DOF)  Controller=PID  Form=Parallel  TimeDomain=Continuous-time  UseExternalTs=off  SampleTime=-1  IntegratorMethod=Forward Euler  FilterMethod=Forward Euler  ControllerParametersSource=internal  P=30  I=20  D=2.5  UseFilter=on  N=100  b=1  c=1  TunerSelectOption=Transfer Function Based (PID Tuner App)  InitialConditionSource=internal  InitialConditionForIntegrator=0  InitialConditionForFilter=0  DifferentiatorICPrevScaledInput=0  ExternalReset=none  TrackingMode=off  Kt=1  LimitOutput=off  SatLimitsSource=internal  UpperSaturationLimit=inf  LowerSaturationLimit=-inf  LinearizeAsGain=on  AntiWindupMode=none  Kb=1  POutMin=[]  POutMax=[]  IOutMin=[]  IOutMax=[]  DOutMin=[]  DOutMax=[]  NOutMin=[]  NOutMax=[]  bOutMin=[]  bOutMax=[]  cOutMin=[]  cOutMax=[]  SumOutMin=[]  SumOutMax=[]  SaturationOutMin=[]  SaturationOutMax=[]  PParamMin=[]  PParamMax=[]  IParamMin=[]  IParamMax=[]  DParamMin=[]  DParamMax=[]  NParamMin=[]  NParamMax=[]  bParamMin=[]  bParamMax=[]  cParamMin=[]  cParamMax=[]  KbParamMin=[]  KbParamMax=[]  KtParamMin=[]  KtParamMax=[]  KbOutMin=[]  KbOutMax=[]  KtOutMin=[]  KtOutMax=[]  IntegratorOutMin=[]  IntegratorOutMax=[]  FilterOutMin=[]  FilterOutMax=[]  SumI1OutMin=[]  SumI1OutMax=[]  SumI2OutMin=[]  SumI2OutMax=[]  SumI3OutMin=[]  SumI3OutMax=[]  SumI4OutMin=[]  SumI4OutMax=[]  SumDOutMin=[]  SumDOutMax=[]  Sum1OutMin=[]  Sum1OutMax=[]  Sum2OutMin=[]  Sum2OutMax=[]  Sum3OutMin=[]  Sum3OutMax=[]  DifferentiatorOutMin=[]  DifferentiatorOutMax=[]  FilterDiffOutCoefMin=[]  FilterDiffOutCoefMax=[]  ReciprocalOutMin=[]  ReciprocalOutMax=[]  SumDenOutMin=[]  SumDenOutMax=[]  SumNumOutMin=[]  SumNumOutMax=[]  DivideOutMin=[]  DivideOutMax=[]  UdiffTsProdOutMin=[]  UdiffTsProdOutMax=[]  NTsProdOutMin=[]  NTsProdOutMax=[]  UintegralTsProdOutMin=[]  UintegralTsProdOutMax=[]  UngainTsProdOutMin=[]  UngainTsProdOutMax=[]  IntegratorContinuousStateAttributes=''  IntegratorStateMustResolveToSignalObject=off  IntegratorRTWStateStorageClass=Auto  FilterContinuousStateAttributes=''  FilterStateMustResolveToSignalObject=off  FilterRTWStateStorageClass=Auto  ParallelPVariant=InternalParameters  IdealPVariant=Disabled  IVariant=InternalParameters  DVariant=InternalParameters  bVariant=InternalParameters  cVariant=InternalParameters  IntegratorVariant=Continuous  SatVariant=Disabled  AWVariant=Passthrough  PCopyVariant=Disabled  TRVariant=Disabled  FdbkBlocksVariant=Forward  IdealPFdbkVariant=Disabled  SatFdbkVariant=Disabled  DerivativeFilterVariant=ContFilter  NVariant=InternalParameters  NCopyVariant=Disabled  FilterICVariant=InternalICsFilter  IntegratorICVariant=InternalICs  ExternalResetVariant=Disabled  TRSumVariant=Passthrough  SumFdbkVariant=Disabled  SumVariant=Sum_PID  TsampFilterVariant=InternalTs  TsampNgainVariant=Passthrough  TsampIntegralVariant=Passthrough  ExternalSaturationOutDataTypeStr=Inherit: Same as second input
      settings: SourceProductBaseCode=SL
  C_q2 : pid_lib/PID Controller (2DOF)  Controller=PID  Form=Parallel  TimeDomain=Continuous-time  UseExternalTs=off  SampleTime=-1  IntegratorMethod=Forward Euler  FilterMethod=Forward Euler  ControllerParametersSource=internal  P=7  I=15  D=0.5  UseFilter=on  N=100  b=1  c=1  TunerSelectOption=Transfer Function Based (PID Tuner App)  InitialConditionSource=internal  InitialConditionForIntegrator=0  InitialConditionForFilter=0  DifferentiatorICPrevScaledInput=0  ExternalReset=none  TrackingMode=off  Kt=1  LimitOutput=off  SatLimitsSource=internal  UpperSaturationLimit=inf  LowerSaturationLimit=-inf  LinearizeAsGain=on  AntiWindupMode=none  Kb=1  POutMin=[]  POutMax=[]  IOutMin=[]  IOutMax=[]  DOutMin=[]  DOutMax=[]  NOutMin=[]  NOutMax=[]  bOutMin=[]  bOutMax=[]  cOutMin=[]  cOutMax=[]  SumOutMin=[]  SumOutMax=[]  SaturationOutMin=[]  SaturationOutMax=[]  PParamMin=[]  PParamMax=[]  IParamMin=[]  IParamMax=[]  DParamMin=[]  DParamMax=[]  NParamMin=[]  NParamMax=[]  bParamMin=[]  bParamMax=[]  cParamMin=[]  cParamMax=[]  KbParamMin=[]  KbParamMax=[]  KtParamMin=[]  KtParamMax=[]  KbOutMin=[]  KbOutMax=[]  KtOutMin=[]  KtOutMax=[]  IntegratorOutMin=[]  IntegratorOutMax=[]  FilterOutMin=[]  FilterOutMax=[]  SumI1OutMin=[]  SumI1OutMax=[]  SumI2OutMin=[]  SumI2OutMax=[]  SumI3OutMin=[]  SumI3OutMax=[]  SumI4OutMin=[]  SumI4OutMax=[]  SumDOutMin=[]  SumDOutMax=[]  Sum1OutMin=[]  Sum1OutMax=[]  Sum2OutMin=[]  Sum2OutMax=[]  Sum3OutMin=[]  Sum3OutMax=[]  DifferentiatorOutMin=[]  DifferentiatorOutMax=[]  FilterDiffOutCoefMin=[]  FilterDiffOutCoefMax=[]  ReciprocalOutMin=[]  ReciprocalOutMax=[]  SumDenOutMin=[]  SumDenOutMax=[]  SumNumOutMin=[]  SumNumOutMax=[]  DivideOutMin=[]  DivideOutMax=[]  UdiffTsProdOutMin=[]  UdiffTsProdOutMax=[]  NTsProdOutMin=[]  NTsProdOutMax=[]  UintegralTsProdOutMin=[]  UintegralTsProdOutMax=[]  UngainTsProdOutMin=[]  UngainTsProdOutMax=[]  IntegratorContinuousStateAttributes=''  IntegratorStateMustResolveToSignalObject=off  IntegratorRTWStateStorageClass=Auto  FilterContinuousStateAttributes=''  FilterStateMustResolveToSignalObject=off  FilterRTWStateStorageClass=Auto  ParallelPVariant=InternalParameters  IdealPVariant=Disabled  IVariant=InternalParameters  DVariant=InternalParameters  bVariant=InternalParameters  cVariant=InternalParameters  IntegratorVariant=Continuous  SatVariant=Disabled  AWVariant=Passthrough  PCopyVariant=Disabled  TRVariant=Disabled  FdbkBlocksVariant=Forward  IdealPFdbkVariant=Disabled  SatFdbkVariant=Disabled  DerivativeFilterVariant=ContFilter  NVariant=InternalParameters  NCopyVariant=Disabled  FilterICVariant=InternalICsFilter  IntegratorICVariant=InternalICs  ExternalResetVariant=Disabled  TRSumVariant=Passthrough  SumFdbkVariant=Disabled  SumVariant=Sum_PID  TsampFilterVariant=InternalTs  TsampNgainVariant=Passthrough  TsampIntegralVariant=Passthrough  ExternalSaturationOutDataTypeStr=Inherit: Same as second input
      settings: SourceProductBaseCode=SL
  Mux1 : Mux  Inputs=2
  Saturate Inputs : Subsystem
  tau : Outport
  wires:
  plant_bus/1 -> [PLANT]
  q_cmd_bus/1 -> [CMD]
  Mux1/1 -> Saturate Inputs/1(inp)
  C_q2/1 -> Mux1/2
  [CMD] -> Bus Selector3/1, Bus Selector/1
  [PLANT] -> Bus Selector2/1, Bus Selector1/1
  Bus Selector1/1 -> C_q1/2  "<q1>"
  Bus Selector2/1 -> C_q2/2  "<q2>"
  Bus Selector3/1 -> C_q2/1  "<cmd_q2>"
  Bus Selector/1 -> C_q1/1  "<cmd_q1>"
  C_q1/1 -> Mux1/1
  Saturate Inputs/1(sat) -> tau/1

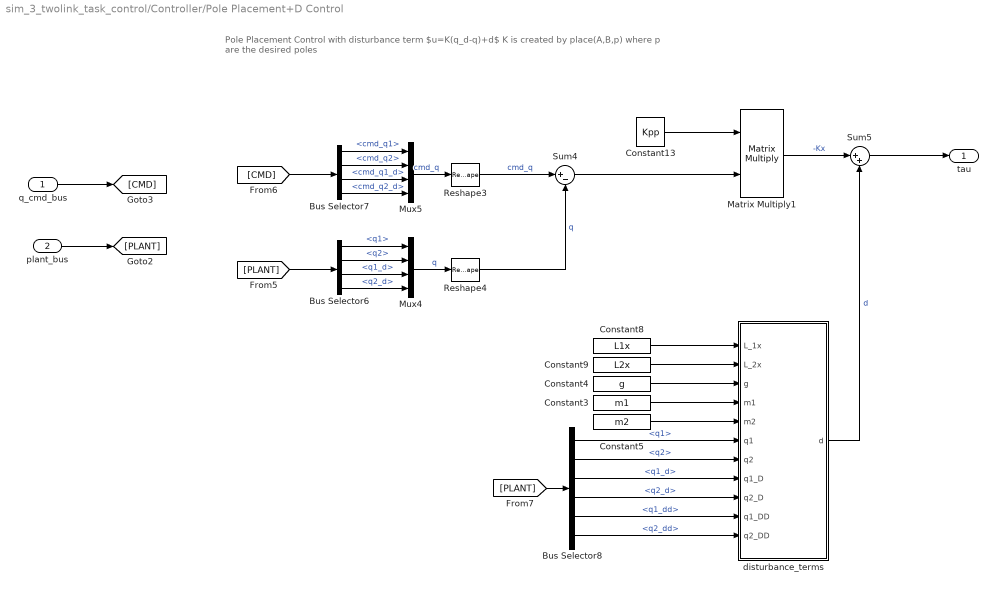
== system sim_3_twolink_task_control/Controller/Pole Placement+D Control ==
  note: Pole Placement Control with disturbance term
      | $u=K(q_d-q)+d$
      | K is created by place(A,B,p) where p are the desired poles
  q_cmd_bus : Inport
  plant_bus : Inport  Port=2
  Bus Selector6 : BusSelector  OutputSignals=q1,q2,q1_d,q2_d
  Bus Selector7 : BusSelector  OutputSignals=cmd_q1,cmd_q2,cmd_q1_d,cmd_q2_d
  Bus Selector8 : BusSelector  OutputSignals=q1,q2,q1_d,q2_d,q1_dd,q2_dd
  Constant13 : Constant  Value=Kpp  VectorParams1D=off
  Constant3 : Constant  Value=m1
  Constant4 : Constant  Value=g
  Constant5 : Constant  Value=m2
  Constant8 : Constant  Value=L1x
  Constant9 : Constant  Value=L2x
  Matrix Multiply1 : Product  Multiplication=Matrix(*)
  Mux4 : Mux
  Mux5 : Mux
  Reshape3 : Reshape  OutputDimensionality=Column vector (2-D)
  Reshape4 : Reshape  OutputDimensionality=Column vector (2-D)
  Sum4 : Sum  Inputs=|+-
  Sum5 : Sum  Inputs=|++
  disturbance_terms : MATLAB Function  TreatAsAtomicUnit=on
  tau : Outport
  wires:
  Bus Selector6/2 -> Mux4/2  "<q2>"
  Bus Selector6/1 -> Mux4/1  "<q1>"
  Mux4/1 -> Reshape4/1  "q"
  q_cmd_bus/1 -> [CMD]
  plant_bus/1 -> [PLANT]
  Mux5/1 -> Reshape3/1  "cmd_q"
  Bus Selector6/3 -> Mux4/3  "<q1_d>"
  [PLANT] -> Bus Selector6/1
  Bus Selector6/4 -> Mux4/4  "<q2_d>"
  Reshape3/1 -> Sum4/1  "cmd_q"
  Reshape4/1 -> Sum4/2  "q"
  Matrix Multiply1/1 -> Sum5/1  "-Kx"
  Sum4/1 -> Matrix Multiply1/2
  Bus Selector7/1 -> Mux5/1  "<cmd_q1>"
  Bus Selector7/2 -> Mux5/2  "<cmd_q2>"
  Bus Selector7/3 -> Mux5/3  "<cmd_q1_d>"
  Constant13/1 -> Matrix Multiply1/1
  Bus Selector7/4 -> Mux5/4  "<cmd_q2_d>"
  [CMD] -> Bus Selector7/1
  Sum5/1 -> tau/1
  disturbance_terms/1(d) -> Sum5/2  "d"
  [PLANT] -> Bus Selector8/1
  Bus Selector8/1 -> disturbance_terms/6(q1)  "<q1>"
  Bus Selector8/2 -> disturbance_terms/7(q2)  "<q2>"
  Bus Selector8/3 -> disturbance_terms/8(q1_D)  "<q1_d>"
  Bus Selector8/4 -> disturbance_terms/9(q2_D)  "<q2_d>"
  Bus Selector8/5 -> disturbance_terms/10(q1_DD)  "<q1_dd>"
  Bus Selector8/6 -> disturbance_terms/11(q2_DD)  "<q2_dd>"
  Constant8/1 -> disturbance_terms/1(L_1x)
  Constant9/1 -> disturbance_terms/2(L_2x)
  Constant4/1 -> disturbance_terms/3(g)
  Constant3/1 -> disturbance_terms/4(m1)
  Constant5/1 -> disturbance_terms/5(m2)

== system sim_3_twolink_task_control/Inverse Kinmatics/Forward Kinmatics ==
  MODEL_BUS : Inport
  Bus Creator : BusCreator  Inputs=2
  Bus Creator1 : BusCreator  Commented=on  Inputs=2
  Bus Selector : BusSelector  OutputSignals=q1,q2
  Constant : Constant  Value=L1x
  Constant1 : Constant  Value=L2x
  Demux3 : Demux  Commented=on  Outputs=3
  Forward Kinematics : MATLAB Function  TreatAsAtomicUnit=on
  Get Transform : robotmaniplib/Get Transform  Commented=on  RigidBodyTree=RR_robot  SourceBody=end_effector  TargetBody=base  SimulateUsing=Interpreted execution
  Mux2 : Mux  Commented=on  Inputs=2
  Reshape : Reshape  Commented=on
  Selector : Selector  Commented=on  InputPortWidth=16  IndexOptions=Index vector (dialog)  Indices=[13:15]  OutputSizes=1
  xy : Outport
  wires:
  Forward Kinematics/2(YE) -> Bus Creator/2  "y"
  Forward Kinematics/1(XE) -> Bus Creator/1  "x"
  Bus Selector/1 -> Mux2/1, Forward Kinematics/3(theta_1)  "<q1>"
  MODEL_BUS/1 -> Bus Selector/1
  Bus Selector/2 -> Mux2/2, Forward Kinematics/4(theta_2)  "<q2>"
  Constant/1 -> Forward Kinematics/1(L_1)
  Constant1/1 -> Forward Kinematics/2(L_2)
  Bus Creator/1 -> xy/1
  Mux2/1 -> Get Transform/1
  Get Transform/1 -> Reshape/1
  Reshape/1 -> Selector/1
  Selector/1 -> Demux3/1
  Demux3/1 -> Bus Creator1/1  "x"
  Demux3/2 -> Bus Creator1/2  "y"

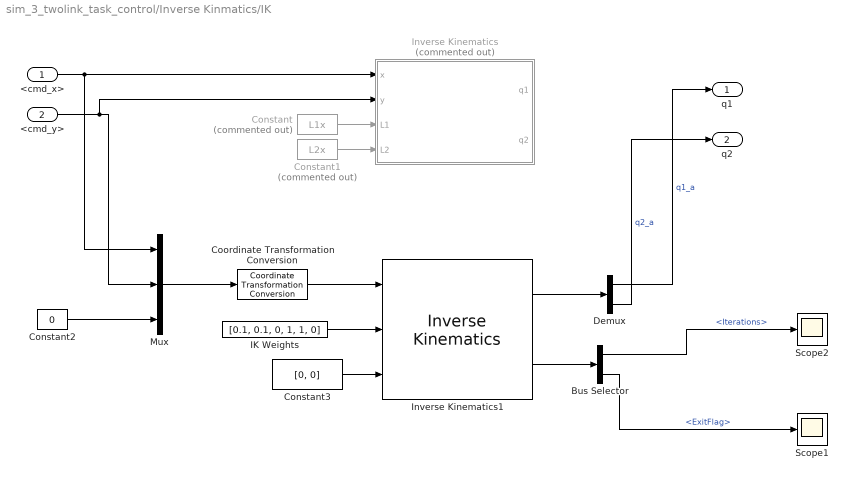
== system sim_3_twolink_task_control/Inverse Kinmatics/IK ==
  <cmd_x> : Inport
  <cmd_y> : Inport  Port=2
  Bus Selector : BusSelector  OutputSignals=Iterations,ExitFlag
  Constant : Constant  Commented=on  Value=L1x
  Constant1 : Constant  Commented=on  Value=L2x
  Constant2 : Constant  Value=0
  Constant3 : Constant  Value=[0, 0]
  Coordinate Transformation Conversion : robotcorelib/Coordinate Transformation Conversion  InputRepresentation=Translation Vector  InputEulerSequence=ZYX  ShowTrVecInputPort=on  OutputRepresentation=Homogeneous Transformation  OutputEulerSequence=ZYX  ShowTrVecOutputPort=on  SimulateUsing=Interpreted execution
      settings: SourceProductBaseCode=RO
  Demux : Demux  Outputs=2
  IK Weights : Constant  Value=[0.1, 0.1, 0, 1, 1, 0]
  Inverse Kinematics : MATLAB Function  Commented=on  TreatAsAtomicUnit=on
  Inverse Kinematics1 : robotmaniplib/Inverse Kinematics  RigidBodyTree=RR_robot  EndEffector=end_effector  ShowInfo=on  SolverName=Levenberg-Marquardt  EnforceJointLimits=on  MaxIterations=30  MaxTime=10  GradientTolerance=1e-7  SolutionTolerance=1e-6  StepTolerance=1e-14  ErrorChangeTolerance=1e-12  UseErrorDamping=on  DampingBias=0.0025  SimulateUsing=Interpreted execution
  Mux : Mux  Inputs=3
  Scope1 : Scope
  Scope2 : Scope
  q1 : Outport
  q2 : Outport  Port=2
  wires:
  Constant1/1 -> Inverse Kinematics/4(L2)
  Constant/1 -> Inverse Kinematics/3(L1)
  <cmd_x>/1 -> Mux/1, Inverse Kinematics/1(x)
  IK Weights/1 -> Inverse Kinematics1/2
  Bus Selector/1 -> Scope2/1  "<Iterations>"
  Inverse Kinematics1/2 -> Bus Selector/1
  Coordinate Transformation Conversion/1 -> Inverse Kinematics1/1
  <cmd_y>/1 -> Inverse Kinematics/2(y), Mux/2
  Constant2/1 -> Mux/3
  Inverse Kinematics1/1 -> Demux/1
  Mux/1 -> Coordinate Transformation Conversion/1
  Bus Selector/2 -> Scope1/1  "<ExitFlag>"
  Constant3/1 -> Inverse Kinematics1/3
  Demux/2 -> q2/1  "q2_a"
  Demux/1 -> q1/1  "q1_a"
